simulink model "ModeloUnicompartimental"  (R2019a)
settings: Solver=VariableStepAuto  StartTime=0.0  StopTime=10.0  RelTol=1e-3
values from neighbouring files (symbols this model uses):
  C = 0.05    [ModeloUnicompartimental_parameters.m]    (also in RLC_parameters.m = 1)
  K = 0.5    [ModeloUnicompartimental_parameters.m]
  Pvent = 20    [ModeloUnicompartimental_parameters.m]
  R = 4    [ModeloUnicompartimental_parameters.m]    (also in RLC_parameters.m = 2)
settings Model: Creator=AnthonyPC  LastModifiedBy=AnthonyPC

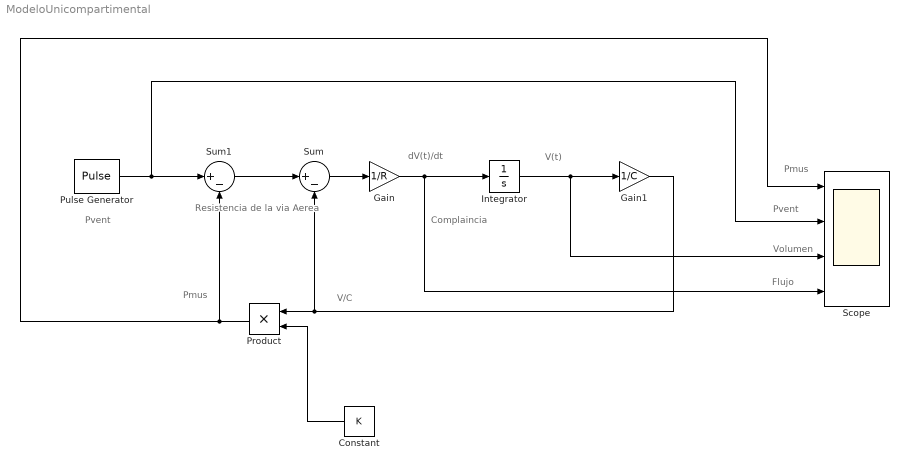
== system ModeloUnicompartimental ==
  note: Flujo
  note: Volumen
  note: Pvent
  note: Pmus
  note: Pmus
  note: V(t)
  note: dV(t)/dt
  note: Resistencia de la via Aerea
  note: Complaincia
  note: V/C
  note: Pvent
  Constant : Constant  Value=K
  Gain : Gain  Gain=1/R
  Gain1 : Gain  Gain=1/C
  Integrator : Integrator
  Product : Product
  Pulse Generator : DiscretePulseGenerator  PulseType=Time based  Amplitude=Pvent  PulseWidth=50
  Scope : Scope  NumInputPorts=4
  Sum : Sum  Inputs=|+-
  Sum1 : Sum  Inputs=|+-
  wires:
  Sum/1 -> Gain/1
  Gain/1 -> Scope/4, Integrator/1
  Integrator/1 -> Gain1/1, Scope/3
  Gain1/1 -> Sum/2, Product/1
  Constant/1 -> Product/2
  Pulse Generator/1 -> Scope/2, Sum1/1
  Product/1 -> Sum1/2, Scope/1
  Sum1/1 -> Sum/1
